simulink model "Aula6_Simulink_v2"  (R2013b)
settings: Solver=ode45  StartTime=0.0  StopTime=10.0  RelTol=1e-3
settings Model: Creator=ThiagoCordeiro  LastModifiedBy=thiag

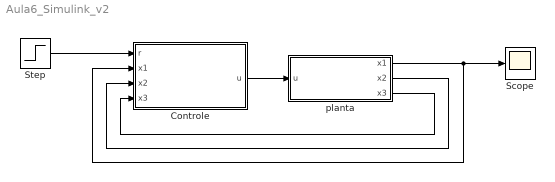
== system Aula6_Simulink_v2 ==
  Controle : Subsystem
  Scope : Scope
  Step : Step  SampleTime=0
  planta : Subsystem
  wires:
  planta/1(x1) -> Controle/2(x1), Scope/1
  Step/1 -> Controle/1(r)
  Controle/1(u) -> planta/1(u)
  planta/3(x3) -> Controle/4(x3)
  planta/2(x2) -> Controle/3(x2)

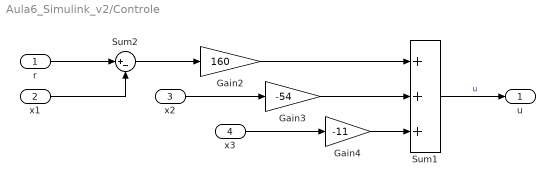
== system Aula6_Simulink_v2/Controle ==
  r : Inport
  x1 : Inport  Port=2
  x2 : Inport  Port=3
  x3 : Inport  Port=4
  Gain2 : Gain  Gain=160
  Gain3 : Gain  Gain=-54
  Gain4 : Gain  Gain=-11
  Sum1 : Sum  Inputs=+++
  Sum2 : Sum  Inputs=|+-
  u : Outport
  wires:
  Gain4/1 -> Sum1/3
  Gain3/1 -> Sum1/2
  Sum2/1 -> Gain2/1
  Gain2/1 -> Sum1/1
  r/1 -> Sum2/1
  Sum1/1 -> u/1  "u"
  x1/1 -> Sum2/2
  x2/1 -> Gain3/1
  x3/1 -> Gain4/1

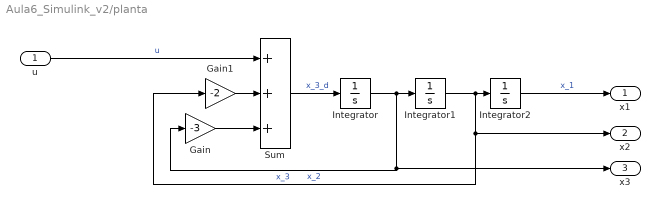
== system Aula6_Simulink_v2/planta ==
  u : Inport
  Gain : Gain  Gain=-3
  Gain1 : Gain  Gain=-2
  Integrator : Integrator
  Integrator1 : Integrator
  Integrator2 : Integrator
  Sum : Sum  Inputs=+++
  x1 : Outport
  x2 : Outport  Port=2
  x3 : Outport  Port=3
  wires:
  Integrator/1 -> Gain/1, x3/1, Integrator1/1  "x_3"
  Integrator1/1 -> Gain1/1, x2/1, Integrator2/1  "x_2"
  Integrator2/1 -> x1/1  "x_1"
  Gain/1 -> Sum/3
  Gain1/1 -> Sum/2
  Sum/1 -> Integrator/1  "x_3_d"
  u/1 -> Sum/1  "u"
